simulink model "generic_mass_and_soc_estimators"  (R2025a)
settings: Solver=ode45  StartTime=0.0  StopTime=inf  RelTol=1e-3  EnableMultiTasking=on
values from neighbouring files (symbols this model uses):
  Battery =     [Battery_A123_Pack_204s2p_Final.mat]
  dOCV_dSoC = gradient(OCV, SoC_bp)    [SoCOcv.m]
  dR0 = gradient(R0, SoC_L)    [SoCOcv.m]
  SoC_bp = Table_SoCvsOCV.LUT.SoC_percent    [SoCOcv.m]
  SoC_L = Battery.SOC_LUT    [SoCOcv.m]
  Table_SoCvsOCV = load("SoC_to_Voltage_LUT_10000-GON.mat")    [SoCOcv.m]
undefined symbols (not defined in the file or in its folder): DiscIntNeverNeededParam
libraries: CarMaker4SL x13, simulink x1
(part 3 of 3)

== system generic_mass_and_soc_estimators/CarMaker/IPG Vehicle/CarAndTrailer/Forces/Suspension Forces/FrcSystem CreateBus CtrlOutOpt ==
  note: <Your model here>
  In : Inport
  Bus Creator9 : BusCreator  Inputs=64
  Demux : Demux  Outputs=64
  Out : Outport
  wires:
  In/1 -> Demux/1
  Bus Creator9/1 -> Out/1
  Demux/64 -> Bus Creator9/64  "CtrlOutOpt63"
  Demux/1 -> Bus Creator9/1  "CtrlOutOpt0"
  Demux/2 -> Bus Creator9/2  "CtrlOutOpt1"
  Demux/3 -> Bus Creator9/3  "CtrlOutOpt2"
  Demux/4 -> Bus Creator9/4  "CtrlOutOpt3"
  Demux/5 -> Bus Creator9/5  "CtrlOutOpt4"
  Demux/6 -> Bus Creator9/6  "CtrlOutOpt5"
  Demux/7 -> Bus Creator9/7  "CtrlOutOpt6"
  Demux/8 -> Bus Creator9/8  "CtrlOutOpt7"
  Demux/9 -> Bus Creator9/9  "CtrlOutOpt8"
  Demux/10 -> Bus Creator9/10  "CtrlOutOpt9"
  Demux/11 -> Bus Creator9/11  "CtrlOutOpt10"
  Demux/12 -> Bus Creator9/12  "CtrlOutOpt11"
  Demux/13 -> Bus Creator9/13  "CtrlOutOpt12"
  Demux/14 -> Bus Creator9/14  "CtrlOutOpt13"
  Demux/15 -> Bus Creator9/15  "CtrlOutOpt14"
  Demux/16 -> Bus Creator9/16  "CtrlOutOpt15"
  Demux/17 -> Bus Creator9/17  "CtrlOutOpt16"
  Demux/18 -> Bus Creator9/18  "CtrlOutOpt17"
  Demux/19 -> Bus Creator9/19  "CtrlOutOpt18"
  Demux/20 -> Bus Creator9/20  "CtrlOutOpt19"
  Demux/21 -> Bus Creator9/21  "CtrlOutOpt20"
  Demux/22 -> Bus Creator9/22  "CtrlOutOpt21"
  Demux/23 -> Bus Creator9/23  "CtrlOutOpt22"
  Demux/24 -> Bus Creator9/24  "CtrlOutOpt23"
  Demux/25 -> Bus Creator9/25  "CtrlOutOpt24"
  Demux/26 -> Bus Creator9/26  "CtrlOutOpt25"
  Demux/27 -> Bus Creator9/27  "CtrlOutOpt26"
  Demux/28 -> Bus Creator9/28  "CtrlOutOpt27"
  Demux/29 -> Bus Creator9/29  "CtrlOutOpt28"
  Demux/30 -> Bus Creator9/30  "CtrlOutOpt29"
  Demux/31 -> Bus Creator9/31  "CtrlOutOpt30"
  Demux/32 -> Bus Creator9/32  "CtrlOutOpt31"
  Demux/33 -> Bus Creator9/33  "CtrlOutOpt32"
  Demux/34 -> Bus Creator9/34  "CtrlOutOpt33"
  Demux/35 -> Bus Creator9/35  "CtrlOutOpt34"
  Demux/36 -> Bus Creator9/36  "CtrlOutOpt35"
  Demux/37 -> Bus Creator9/37  "CtrlOutOpt36"
  Demux/38 -> Bus Creator9/38  "CtrlOutOpt37"
  Demux/39 -> Bus Creator9/39  "CtrlOutOpt38"
  Demux/40 -> Bus Creator9/40  "CtrlOutOpt39"
  Demux/41 -> Bus Creator9/41  "CtrlOutOpt40"
  Demux/42 -> Bus Creator9/42  "CtrlOutOpt41"
  Demux/43 -> Bus Creator9/43  "CtrlOutOpt42"
  Demux/44 -> Bus Creator9/44  "CtrlOutOpt43"
  Demux/45 -> Bus Creator9/45  "CtrlOutOpt44"
  Demux/46 -> Bus Creator9/46  "CtrlOutOpt45"
  Demux/47 -> Bus Creator9/47  "CtrlOutOpt46"
  Demux/48 -> Bus Creator9/48  "CtrlOutOpt47"
  Demux/49 -> Bus Creator9/49  "CtrlOutOpt48"
  Demux/50 -> Bus Creator9/50  "CtrlOutOpt49"
  Demux/51 -> Bus Creator9/51  "CtrlOutOpt50"
  Demux/52 -> Bus Creator9/52  "CtrlOutOpt51"
  Demux/53 -> Bus Creator9/53  "CtrlOutOpt52"
  Demux/54 -> Bus Creator9/54  "CtrlOutOpt53"
  Demux/55 -> Bus Creator9/55  "CtrlOutOpt54"
  Demux/56 -> Bus Creator9/56  "CtrlOutOpt55"
  Demux/57 -> Bus Creator9/57  "CtrlOutOpt56"
  Demux/58 -> Bus Creator9/58  "CtrlOutOpt57"
  Demux/59 -> Bus Creator9/59  "CtrlOutOpt58"
  Demux/60 -> Bus Creator9/60  "CtrlOutOpt59"
  Demux/61 -> Bus Creator9/61  "CtrlOutOpt60"
  Demux/62 -> Bus Creator9/62  "CtrlOutOpt61"
  Demux/63 -> Bus Creator9/63  "CtrlOutOpt62"

== system generic_mass_and_soc_estimators/CarMaker/IPG Vehicle/CarAndTrailer/Forces/Suspension Forces/Spring CreateBus CtrlOutOpt ==
  note: <Your model here>
  In : Inport
  Bus Creator{,1..3,9} (5 alike) : BusCreator  Inputs=4
  Demux{,2..5} (5 alike) : Demux
  Out : Outport
  wires:
  Bus Creator/1 -> Bus Creator9/1
  Demux/4 -> Demux5/1  "RR"
  Bus Creator2/1 -> Bus Creator9/3
  Demux5/1 -> Bus Creator3/1  "RR CtrlOutOpt0"
  Bus Creator3/1 -> Bus Creator9/4
  Demux2/4 -> Bus Creator/4  "FL CtrlOutOpt3"
  Demux5/3 -> Bus Creator3/3  "RR CtrlOutOpt2"
  Demux4/3 -> Bus Creator2/3  "RL CtrlOutOpt2"
  Bus Creator1/1 -> Bus Creator9/2
  Demux4/2 -> Bus Creator2/2  "RL CtrlOutOpt1"
  Demux2/2 -> Bus Creator/2  "FL CtrlOutOpt1"
  Demux/2 -> Demux3/1  "FR"
  Demux3/4 -> Bus Creator1/4  "FR CtrlOutOpt3"
  Demux3/1 -> Bus Creator1/1  "FR CtrlOutOpt0"
  Demux4/4 -> Bus Creator2/4  "RL CtrlOutOpt3"
  Demux2/3 -> Bus Creator/3  "FL CtrlOutOpt2"
  Demux3/2 -> Bus Creator1/2  "FR CtrlOutOpt1"
  Demux2/1 -> Bus Creator/1  "FL CtrlOutOpt0"
  Demux3/3 -> Bus Creator1/3  "FR CtrlOutOpt2"
  In/1 -> Demux/1
  Demux5/4 -> Bus Creator3/4  "RR CtrlOutOpt3"
  Demux/3 -> Demux4/1  "RL"
  Bus Creator9/1 -> Out/1
  Demux5/2 -> Bus Creator3/2  "RR CtrlOutOpt1"
  Demux4/1 -> Bus Creator2/1  "RL CtrlOutOpt0"
  Demux/1 -> Demux2/1  "FL"

== system generic_mass_and_soc_estimators/CarMaker/IPG Vehicle/CarAndTrailer/Forces/Suspension Forces/Stabi CreateBus CtrlOutOpt ==
  note: <Your model here>
  In : Inport
  Bus Creator{,1..3,9} (5 alike) : BusCreator  Inputs=4
  Demux{,2..5} (5 alike) : Demux
  Out : Outport
  wires:
  Bus Creator/1 -> Bus Creator9/1
  Demux/4 -> Demux5/1  "RR"
  Bus Creator2/1 -> Bus Creator9/3
  Demux5/1 -> Bus Creator3/1  "RR CtrlOutOpt0"
  Bus Creator3/1 -> Bus Creator9/4
  Demux2/4 -> Bus Creator/4  "FL CtrlOutOpt3"
  Demux5/3 -> Bus Creator3/3  "RR CtrlOutOpt2"
  Demux4/3 -> Bus Creator2/3  "RL CtrlOutOpt2"
  Bus Creator1/1 -> Bus Creator9/2
  Demux4/2 -> Bus Creator2/2  "RL CtrlOutOpt1"
  Demux2/2 -> Bus Creator/2  "FL CtrlOutOpt1"
  Demux/2 -> Demux3/1  "FR"
  Demux3/4 -> Bus Creator1/4  "FR CtrlOutOpt3"
  Demux3/1 -> Bus Creator1/1  "FR CtrlOutOpt0"
  Demux4/4 -> Bus Creator2/4  "RL CtrlOutOpt3"
  Demux2/3 -> Bus Creator/3  "FL CtrlOutOpt2"
  Demux3/2 -> Bus Creator1/2  "FR CtrlOutOpt1"
  Demux2/1 -> Bus Creator/1  "FL CtrlOutOpt0"
  Demux3/3 -> Bus Creator1/3  "FR CtrlOutOpt2"
  In/1 -> Demux/1
  Demux5/4 -> Bus Creator3/4  "RR CtrlOutOpt3"
  Demux/3 -> Demux4/1  "RL"
  Bus Creator9/1 -> Out/1
  Demux5/2 -> Bus Creator3/2  "RR CtrlOutOpt1"
  Demux4/1 -> Bus Creator2/1  "RL CtrlOutOpt0"
  Demux/1 -> Demux2/1  "FL"

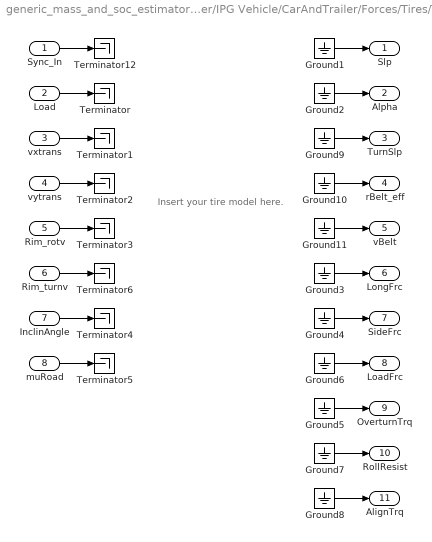
== system generic_mass_and_soc_estimators/CarMaker/IPG Vehicle/CarAndTrailer/Forces/Tires/TireFL ==
  note: Insert your tire model here.
  Sync_In : Inport
  Load : Inport  Port=2
  vxtrans : Inport  Port=3
  vytrans : Inport  Port=4
  Rim_rotv : Inport  Port=5
  Rim_turnv : Inport  Port=6
  InclinAngle : Inport  Port=7
  muRoad : Inport  Port=8
  Ground{1..11} (11 alike) : Ground
  Terminator{,1..6,12} (8 alike) : Terminator
  Slp : Outport  VectorParamsAs1DForOutWhenUnconnected=off
  Alpha : Outport  Port=2  VectorParamsAs1DForOutWhenUnconnected=off
  TurnSlp : Outport  Port=3  VectorParamsAs1DForOutWhenUnconnected=off
  rBelt_eff : Outport  Port=4  VectorParamsAs1DForOutWhenUnconnected=off
  vBelt : Outport  Port=5  VectorParamsAs1DForOutWhenUnconnected=off
  LongFrc : Outport  Port=6  VectorParamsAs1DForOutWhenUnconnected=off
  SideFrc : Outport  Port=7  VectorParamsAs1DForOutWhenUnconnected=off
  LoadFrc : Outport  Port=8  VectorParamsAs1DForOutWhenUnconnected=off
  OverturnTrq : Outport  Port=9  VectorParamsAs1DForOutWhenUnconnected=off
  RollResist : Outport  Port=10  VectorParamsAs1DForOutWhenUnconnected=off
  AlignTrq : Outport  Port=11  VectorParamsAs1DForOutWhenUnconnected=off
  wires:
  Ground11/1 -> vBelt/1
  Ground10/1 -> rBelt_eff/1
  Ground9/1 -> TurnSlp/1
  Rim_turnv/1 -> Terminator6/1
  Sync_In/1 -> Terminator12/1
  Ground2/1 -> Alpha/1
  Ground3/1 -> LongFrc/1
  Ground4/1 -> SideFrc/1
  Ground5/1 -> OverturnTrq/1
  vxtrans/1 -> Terminator1/1
  vytrans/1 -> Terminator2/1
  Rim_rotv/1 -> Terminator3/1
  InclinAngle/1 -> Terminator4/1
  muRoad/1 -> Terminator5/1
  Load/1 -> Terminator/1
  Ground1/1 -> Slp/1
  Ground6/1 -> LoadFrc/1
  Ground7/1 -> RollResist/1
  Ground8/1 -> AlignTrq/1

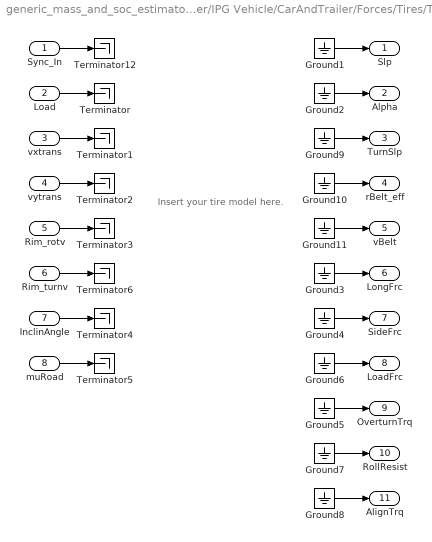
== system generic_mass_and_soc_estimators/CarMaker/IPG Vehicle/CarAndTrailer/Forces/Tires/TireFR ==
  note: Insert your tire model here.
  Sync_In : Inport
  Load : Inport  Port=2
  vxtrans : Inport  Port=3
  vytrans : Inport  Port=4
  Rim_rotv : Inport  Port=5
  Rim_turnv : Inport  Port=6
  InclinAngle : Inport  Port=7
  muRoad : Inport  Port=8
  Ground{1..11} (11 alike) : Ground
  Terminator{,1..6,12} (8 alike) : Terminator
  Slp : Outport  VectorParamsAs1DForOutWhenUnconnected=off
  Alpha : Outport  Port=2  VectorParamsAs1DForOutWhenUnconnected=off
  TurnSlp : Outport  Port=3  VectorParamsAs1DForOutWhenUnconnected=off
  rBelt_eff : Outport  Port=4  VectorParamsAs1DForOutWhenUnconnected=off
  vBelt : Outport  Port=5  VectorParamsAs1DForOutWhenUnconnected=off
  LongFrc : Outport  Port=6  VectorParamsAs1DForOutWhenUnconnected=off
  SideFrc : Outport  Port=7  VectorParamsAs1DForOutWhenUnconnected=off
  LoadFrc : Outport  Port=8  VectorParamsAs1DForOutWhenUnconnected=off
  OverturnTrq : Outport  Port=9  VectorParamsAs1DForOutWhenUnconnected=off
  RollResist : Outport  Port=10  VectorParamsAs1DForOutWhenUnconnected=off
  AlignTrq : Outport  Port=11  VectorParamsAs1DForOutWhenUnconnected=off
  wires:
  Ground11/1 -> vBelt/1
  Ground10/1 -> rBelt_eff/1
  Ground9/1 -> TurnSlp/1
  Rim_turnv/1 -> Terminator6/1
  Sync_In/1 -> Terminator12/1
  Ground2/1 -> Alpha/1
  Ground3/1 -> LongFrc/1
  Ground4/1 -> SideFrc/1
  Ground5/1 -> OverturnTrq/1
  vxtrans/1 -> Terminator1/1
  vytrans/1 -> Terminator2/1
  Rim_rotv/1 -> Terminator3/1
  InclinAngle/1 -> Terminator4/1
  muRoad/1 -> Terminator5/1
  Load/1 -> Terminator/1
  Ground1/1 -> Slp/1
  Ground6/1 -> LoadFrc/1
  Ground7/1 -> RollResist/1
  Ground8/1 -> AlignTrq/1

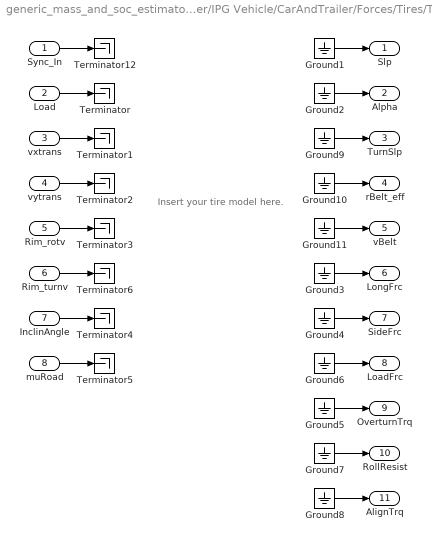
== system generic_mass_and_soc_estimators/CarMaker/IPG Vehicle/CarAndTrailer/Forces/Tires/TireRL ==
  note: Insert your tire model here.
  Sync_In : Inport
  Load : Inport  Port=2
  vxtrans : Inport  Port=3
  vytrans : Inport  Port=4
  Rim_rotv : Inport  Port=5
  Rim_turnv : Inport  Port=6
  InclinAngle : Inport  Port=7
  muRoad : Inport  Port=8
  Ground{1..11} (11 alike) : Ground
  Terminator{,1..6,12} (8 alike) : Terminator
  Slp : Outport  VectorParamsAs1DForOutWhenUnconnected=off
  Alpha : Outport  Port=2  VectorParamsAs1DForOutWhenUnconnected=off
  TurnSlp : Outport  Port=3  VectorParamsAs1DForOutWhenUnconnected=off
  rBelt_eff : Outport  Port=4  VectorParamsAs1DForOutWhenUnconnected=off
  vBelt : Outport  Port=5  VectorParamsAs1DForOutWhenUnconnected=off
  LongFrc : Outport  Port=6  VectorParamsAs1DForOutWhenUnconnected=off
  SideFrc : Outport  Port=7  VectorParamsAs1DForOutWhenUnconnected=off
  LoadFrc : Outport  Port=8  VectorParamsAs1DForOutWhenUnconnected=off
  OverturnTrq : Outport  Port=9  VectorParamsAs1DForOutWhenUnconnected=off
  RollResist : Outport  Port=10  VectorParamsAs1DForOutWhenUnconnected=off
  AlignTrq : Outport  Port=11  VectorParamsAs1DForOutWhenUnconnected=off
  wires:
  Ground11/1 -> vBelt/1
  Ground10/1 -> rBelt_eff/1
  Ground9/1 -> TurnSlp/1
  Rim_turnv/1 -> Terminator6/1
  Sync_In/1 -> Terminator12/1
  Ground2/1 -> Alpha/1
  Ground3/1 -> LongFrc/1
  Ground4/1 -> SideFrc/1
  Ground5/1 -> OverturnTrq/1
  vxtrans/1 -> Terminator1/1
  vytrans/1 -> Terminator2/1
  Rim_rotv/1 -> Terminator3/1
  InclinAngle/1 -> Terminator4/1
  muRoad/1 -> Terminator5/1
  Load/1 -> Terminator/1
  Ground1/1 -> Slp/1
  Ground6/1 -> LoadFrc/1
  Ground7/1 -> RollResist/1
  Ground8/1 -> AlignTrq/1

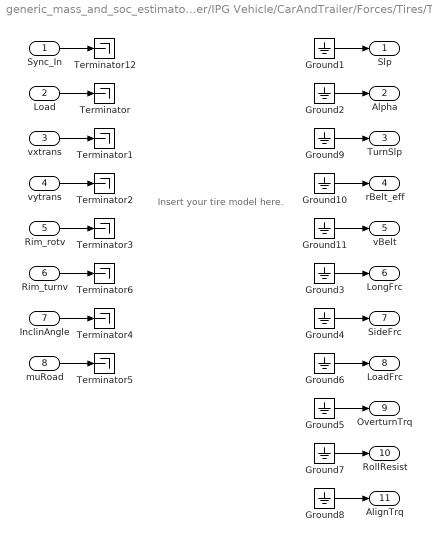
== system generic_mass_and_soc_estimators/CarMaker/IPG Vehicle/CarAndTrailer/Forces/Tires/TireRR ==
  note: Insert your tire model here.
  Sync_In : Inport
  Load : Inport  Port=2
  vxtrans : Inport  Port=3
  vytrans : Inport  Port=4
  Rim_rotv : Inport  Port=5
  Rim_turnv : Inport  Port=6
  InclinAngle : Inport  Port=7
  muRoad : Inport  Port=8
  Ground{1..11} (11 alike) : Ground
  Terminator{,1..6,12} (8 alike) : Terminator
  Slp : Outport  VectorParamsAs1DForOutWhenUnconnected=off
  Alpha : Outport  Port=2  VectorParamsAs1DForOutWhenUnconnected=off
  TurnSlp : Outport  Port=3  VectorParamsAs1DForOutWhenUnconnected=off
  rBelt_eff : Outport  Port=4  VectorParamsAs1DForOutWhenUnconnected=off
  vBelt : Outport  Port=5  VectorParamsAs1DForOutWhenUnconnected=off
  LongFrc : Outport  Port=6  VectorParamsAs1DForOutWhenUnconnected=off
  SideFrc : Outport  Port=7  VectorParamsAs1DForOutWhenUnconnected=off
  LoadFrc : Outport  Port=8  VectorParamsAs1DForOutWhenUnconnected=off
  OverturnTrq : Outport  Port=9  VectorParamsAs1DForOutWhenUnconnected=off
  RollResist : Outport  Port=10  VectorParamsAs1DForOutWhenUnconnected=off
  AlignTrq : Outport  Port=11  VectorParamsAs1DForOutWhenUnconnected=off
  wires:
  Ground11/1 -> vBelt/1
  Ground10/1 -> rBelt_eff/1
  Ground9/1 -> TurnSlp/1
  Rim_turnv/1 -> Terminator6/1
  Sync_In/1 -> Terminator12/1
  Ground2/1 -> Alpha/1
  Ground3/1 -> LongFrc/1
  Ground4/1 -> SideFrc/1
  Ground5/1 -> OverturnTrq/1
  vxtrans/1 -> Terminator1/1
  vytrans/1 -> Terminator2/1
  Rim_rotv/1 -> Terminator3/1
  InclinAngle/1 -> Terminator4/1
  muRoad/1 -> Terminator5/1
  Load/1 -> Terminator/1
  Ground1/1 -> Slp/1
  Ground6/1 -> LoadFrc/1
  Ground7/1 -> RollResist/1
  Ground8/1 -> AlignTrq/1

== matlab function generic_mass_and_soc_estimators/CarMaker/MATLAB Function3 ==
  data: T_tq input; phi output; vx input; re input
function phi = compute_phi(T_tq, vx, re)

eta=0.95;

rho = 1.225;
Cd  = 0.29;
A   = 2.45;

F_trac = (T_tq*eta) / re;
F_aero = 0.5 * Cd * A * rho * vx * vx;

phi = F_trac - F_aero;

== matlab function generic_mass_and_soc_estimators/CarMaker/Slope estimator ==
  settings: updateMethod=DISCRETE
  data: y2 input; theta2_hat output; phi2 input; lambda2 input; reset2 input; beta_hat output; P2_out output; L2_out output; eps2_out output; t input
function [theta2_hat, beta_hat, P2_out, L2_out, eps2_out] = slope_rls(y2, phi2, lambda2, reset2, t)

    persistent theta2 P2 initialized2

    if isempty(initialized2) || reset2
        theta2 = 0;    % Initial guess for slope-related parameter
        P2 = 1e6;      % Large initial covariance
        initialized2 = true;
    end

    % Hold estimator during first second
    if t < 5
        theta2_hat = theta2;
        beta_hat   = theta2;
        P2_out     = P2;
        L2_out     = 0;
        eps2_out   = 0;
        return
    end

    % Prediction error
    eps2 = y2 - phi2 * theta2;

    % RLS gain
    L2 = (P2 * phi2) / (lambda2 + phi2 * P2 * phi2);

    % Parameter update
    theta2 = theta2 + L2 * eps2;

    % Covariance update
    P2 = (P2 * (1 - L2 * phi2)) / lambda2;

    % Outputs
    theta2_hat = theta2;
    beta_hat   = theta2_hat;

    P2_out   = P2;
    L2_out   = L2;
    eps2_out = eps2;
end

== matlab function generic_mass_and_soc_estimators/CarMaker/MATLAB Function5 ==
  data: Tq input; y2 output; vx input; mhat input; ax input; re input
function y2 = compute_y2(Tq, vx, mhat,ax, re)

eta=0.95;

rho = 1.225;
Cd  = 0.29;
g= 9.81;
A   = 2.45;
f=0.015;
F_aero = 0.5 * Cd * A * rho * vx * vx;
F_rolling = mhat * g * f;

y2 = (Tq)*eta/re -F_aero - F_rolling- mhat * ax;

== matlab function generic_mass_and_soc_estimators/CarMaker/MATLAB Function6 ==
  data: mhat input; phi2 output
function phi2 = compute_phi2(mhat)
g=9.81;

phi2 = mhat * g;

== matlab function generic_mass_and_soc_estimators/CarMaker/COLOUMB COUNTING/MATLAB Function2 ==
  data: Ct input; SoC output; SOC_init input; I input
function SoC = fcn(Ct,SOC_init,I)

% Ct : Battery total capacity (mAh)
% SOC_init : Initial SoC (%)
% I : Cumulative Current (used capacity in mAh)
% y : SoC

 SoC = SOC_init - 100*(I/Ct) ;

end

== matlab function generic_mass_and_soc_estimators/CarMaker/MATLAB Function ==
  data: R_batt input; C_batt output; R_init input; C_init input
function C_batt = capacity_from_r0_linear(R_batt, R_init, C_init)
    C_init=C_init/1000;

    if R_init <= 0
        R_init = 1e-6;
    end

    C_batt = C_init * (1 - 0.2 * (R_batt - R_init) / R_init);

    if C_batt > C_init
        C_batt = C_init;
    elseif C_batt < 0.8 * C_init
        C_batt = 0.8 * C_init;
    end
end

== matlab function generic_mass_and_soc_estimators/CarMaker/EKF ==
  settings: updateMethod=DISCRETE
  data: I input; soc_hat output; UL_meas input; Uoc input; R0_est input; R0nom input; R1 input; C1 input; dUoc_dSoc input; reset input; u1_hat output; ul_hat output; innov output; K_out output; P_out output; Qcap_est input; Qnom input
function [soc_hat, u1_hat, ul_hat, innov, K_out, P_out] = ...
    soc_ekf_paper_1rc(I, UL_meas, Uoc, R0_est, R0nom, R1, C1, dUoc_dSoc, reset, Qcap_est,Qnom)

    persistent x_hat P initialized

    Dt   = 0.01;
    Qnom = 3.6*Qnom;
    Qcap_est = Qcap_est*3600;
    

    Rekf = 1e-1;

    if isempty(initialized) || reset
        x_hat = [0.8;
                 0.0];

        P = [1e-6, 0;
             0,    1e-6];

        initialized = true;
    end

    
    if Qcap_est > 0
        Q0 = Qcap_est;
    else
        Q0 = Qnom;
    end

    
    if R0_est > 1e-3
        R0 = R0_est;
    else
        R0 = R0nom;
    end

    tau1 = R1 * C1;
    a1 = exp(-Dt / tau1);

    A = [1,  0;
         0, a1];

    B = [-Dt / Q0;
         R1 * (1 - exp(-Dt / tau1))];

    sigma_I2 = 1e-1;
    Q_input  = (B * B.') * sigma_I2;

    Q_base = [1e-8, 0;
              0,    1e-8];

    Qekf = Q_base + Q_input;

    % (1) State prediction
    x_pred = A * x_hat + B * I;

    % (2) Covariance prediction
    P_pred = A * P * A.' + Qekf;

    % (3) Measurement Jacobian
    C = [dUoc_dSoc, -1];

    % (4) Predicted output
    ul_hat = Uoc - R0 * I - x_pred(2);

    % (5) Kalman gain
    S = C * P_pred * C.' + Rekf;
    K = (P_pred * C.') / S;

    % (6) State update
    innov = UL_meas - ul_hat;
    x_hat = x_pred + K * innov;

    % (7) Covariance update
    I2 = eye(2);
    P = (I2 - K * C) * P_pred;

    % Outputs
    soc_hat = x_hat(1);
    u1_hat  = x_hat(2);
    K_out   = K;
    P_out   = P;
end

== matlab function generic_mass_and_soc_estimators/CarMaker/RC network subsystem/MATLAB Function ==
  data: I input; y output; R1 input; C1 input; V1 input
function y = fcn(I,R1,C1,V1)

y = -V1/(R1*C1)+I/C1;

== matlab function generic_mass_and_soc_estimators/CarMaker/Mass Estimator ==
  settings: updateMethod=DISCRETE
  data: y input; phi input; lambda input; m_hat output; t input; ax input
function m_hat = mass_rls(y, phi, lambda, t, ax)
    persistent theta P initialized t_start est_active done
    if isempty(initialized)
        theta = 1/2200;
        P = 1e6;
        t_start = 0;
        est_active = false;
        done = false;
        initialized = true;
    end
    theta_min = 1/3000;
    theta_max = 1/1500;
   
    if ~done && ~est_active && abs(ax) > 0.5
        est_active = true;
        t_start = t;
    end
   
    if est_active
        if (t - t_start) <= 10
            eps = y - phi * theta;
            L = (P * phi) / (lambda + phi * P * phi);
            theta = theta + L * eps;
            P = (P * (1 - L * phi)) / lambda;
            if theta < theta_min
                theta = theta_min;
            elseif theta > theta_max
                theta = theta_max;
            end
        else
            est_active = false;
            done = true;
        end
    end
    m_hat = 1 / theta;
end

== matlab function generic_mass_and_soc_estimators/CarMaker/MATLAB Function2 ==
  data: ax input; y output; beta input
function y = compute_y(ax,beta) 
g=9.81; 
f=0.015; 
delta=1; 
y = delta*ax + g*f + g*sin(beta);

== matlab function generic_mass_and_soc_estimators/CarMaker/INTERNAL RESISTANCE ESTIMATION ==
  settings: updateMethod=DISCRETE
  data: I input; R0_hat output; UL_meas input; Uoc input; R0_init input; u1_hat input; reset input; innov_theta output; Ktheta_out output; Ptheta_out output
function [R0_hat, innov_theta, Ktheta_out, Ptheta_out] = ...
    r0_ekf_simple(I, UL_meas, Uoc, R0_init, u1_hat, reset)

    persistent theta_hat Ptheta initialized

    % theta = R0
    Qtheta = 1e-10;
    Rtheta = 1e-1;

    if isempty(initialized) || reset
        theta_hat = R0_init;
        Ptheta = 1e-4;
        initialized = true;
    end
    % (1) PARAMETER PREDICTION
    theta_pred  = theta_hat;
    Ptheta_pred = Ptheta + Qtheta;
    R0_pred = theta_pred;
    % (2) PARAMETER JACOBIAN
    % UL = Uoc - R0*I - U1
    % d(UL)/d(R0) = -I
    Htheta = -I;
    % (3) OUTPUT PREDICTION
    ul_hat_theta = Uoc - R0_pred * I - u1_hat;
    innov_theta = UL_meas - ul_hat_theta;
    % (4) KALMAN GAIN
    S_theta = Htheta * Ptheta_pred * Htheta' + Rtheta;
    Ktheta = (Ptheta_pred * Htheta') / S_theta;
    % (5) PARAMETER UPDATE
    theta_hat = theta_pred + Ktheta * innov_theta;
    % (6) COVARIANCE UPDATE
    Ptheta = (1 - Ktheta * Htheta) * Ptheta_pred;
    % Outputs
    R0_hat = theta_hat;
    Ktheta_out = Ktheta;
    Ptheta_out = Ptheta;

end

== matlab function generic_mass_and_soc_estimators/CarMaker/COLOUMB COUNTING/MATLAB Function1 ==
  data: Ct input; SoC output; SOC_init input; I input
function SoC = fcn(Ct,SOC_init,I)

% Ct : Battery total capacity (mAh)
% SOC_init : Initial SoC (%)
% I : Cumulative Current (used capacity in mAh)
% y : SoC

 SoC = SOC_init - 100*(I/Ct) ;

end

== matlab function generic_mass_and_soc_estimators/CarMaker/MATLAB Function4 ==
  data: Qmax input; Q_real output; factor_internal_resistance input
function Q_real = fcn(Qmax,factor_internal_resistance)

Q_real=Qmax*(1-0.2*(factor_internal_resistance-1));
